simulink model "PI_Laengsregler"  (R2019b)
settings: Solver=FixedStepAuto  StartTime=0.0  StopTime=20  FixedStep=1e-6  RelTol=1e-3
values from neighbouring files (symbols this model uses):
  A = [0, 1;-f(1), -f(2)]    [init.m]    (also in matlab.mat = [0  1; -39.4784176044  -8.88576587632])
  b = [0; 1]    [init.m]    (also in matlab.mat = [0 1])
  cT = [f(1), 0]    [init.m]    (also in matlab.mat = [39.4784176044 0])
  ir = 1.7    [init.m]    (also in matlab.mat)
  pr = 1.3    [init.m]    (also in matlab.mat)
  tau = 3.215/5    (= 0.643)    [init.m]    (also in matlab.mat)
  Ur = pi*0.056    (= 0.175929188601)    [init.m]    (also in matlab.mat)
  v = 2    [init.m]    (also in matlab.mat)
libraries: robotlib x4, simulink x1, cstblocks x1

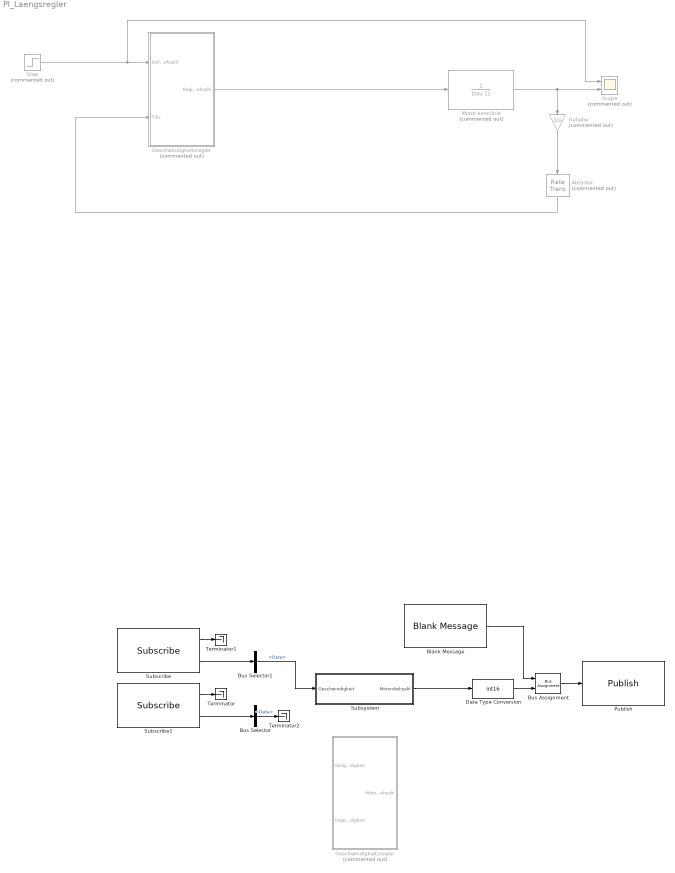
== system PI_Laengsregler ==
  Abtaster : RateTransition  Commented=on  OutPortSampleTime=tasten
  Blank Message : robotlib/Blank Message  messageClass=Message  entityType=std_msgs/Int16  messageType=std_msgs/Int16  SampleTime=inf
  Bus Assignment : BusAssignment  AssignedSignals=Data
  Bus Selector : BusSelector  OutputSignals=Data
  Bus Selector1 : BusSelector  OutputSignals=Data
  Data Type Conversion : DataTypeConversion  OutDataTypeStr=int16
  Geschwindigkeitsregler : Subsystem  Commented=on
  "Geschwindigkeitsregler " : Subsystem  Commented=on
  Getiebe : Gain  Commented=on  Gain=1/u
  Motor kennlinie : TransferFcn  Commented=on  Denominator=[tau 1]
  Publish : robotlib/Publish  topicSource=Specify your own  topic=/ctl_motorRpm  messageType=std_msgs/Int16  messageQueueLength=1
  Scope : Scope  Commented=on  NumInputPorts=2
  Step : Step  Commented=on  After=u*v/Ur  SampleTime=0
  Subscribe : robotlib/Subscribe  topicSource=Specify your own  topic=/trj_targetSpeed  messageType=std_msgs/Float32  sampleTime=-1  messageQueueLength=1
  Subscribe1 : robotlib/Subscribe  topicSource=Specify your own  topic=/ctl_velocity  messageType=std_msgs/Float32  sampleTime=-1  messageQueueLength=1
  Subsystem : Subsystem
  Terminator : Terminator
  Terminator1 : Terminator
  Terminator2 : Terminator
  wires:
  Getiebe/1 -> Abtaster/1
  Motor kennlinie/1 -> Getiebe/1, Scope/2
  Step/1 -> Scope/1, "Geschwindigkeitsregler "/1("Sollmotordrehzahl ")
  "Geschwindigkeitsregler "/1(Reglermotordrehzahl) -> Motor kennlinie/1
  Abtaster/1 -> "Geschwindigkeitsregler "/2(Tiks)
  Subscribe/2 -> Bus Selector1/1
  Subscribe1/2 -> Bus Selector/1
  Bus Assignment/1 -> Publish/1
  Blank Message/1 -> Bus Assignment/1
  Data Type Conversion/1 -> Bus Assignment/2
  Subscribe1/1 -> Terminator/1
  Subscribe/1 -> Terminator1/1
  Bus Selector1/1 -> Subsystem/1(Geschwindigkeit)  "<Data>"
  Subsystem/1(Motordrehzahl) -> Data Type Conversion/1
  Bus Selector/1 -> Terminator2/1  "<Data>"

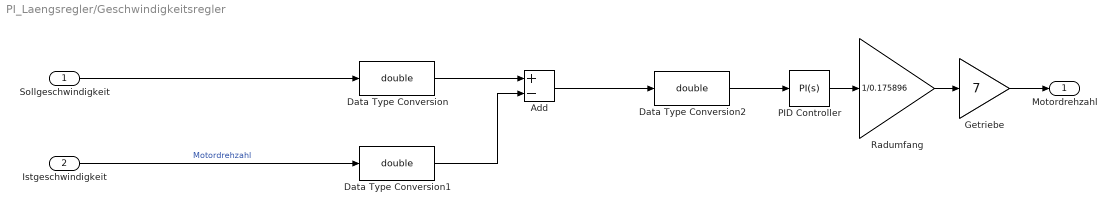
== system PI_Laengsregler/Geschwindigkeitsregler ==
  "Sollgeschwindigkeit " : Inport
  "Istgeschwindigkeit " : Inport  Port=2
  Add : Sum  Inputs=+-
  Data Type Conversion : DataTypeConversion  OutDataTypeStr=double
  Data Type Conversion1 : DataTypeConversion  OutDataTypeStr=double
  Data Type Conversion2 : DataTypeConversion  OutDataTypeStr=double
  Getriebe : Gain  Gain=7
  PID Controller : simulink/Continuous/PID Controller  Controller=PI  Form=Parallel  TimeDomain=Continuous-time  SampleTime=-1  IntegratorMethod=Forward Euler  FilterMethod=Forward Euler  ControllerParametersSource=internal  P=pr  I=ir  D=0  UseFilter=on  N=100  TunerSelectOption=Transfer Function Based (PID Tuner App)  InitialConditionSource=internal  InitialConditionForIntegrator=0  InitialConditionForFilter=0  DifferentiatorICPrevScaledInput=0  ExternalReset=none  TrackingMode=off  Kt=1  LimitOutput=off  UpperSaturationLimit=inf  LowerSaturationLimit=-inf  LinearizeAsGain=on  AntiWindupMode=none  Kb=1  POutMin=[]  POutMax=[]  IOutMin=[]  IOutMax=[]  DOutMin=[]  DOutMax=[]  NOutMin=[]  NOutMax=[]  SumOutMin=[]  SumOutMax=[]  SaturationOutMin=[]  SaturationOutMax=[]  PParamMin=[]  PParamMax=[]  IParamMin=[]  IParamMax=[]  DParamMin=[]  DParamMax=[]  NParamMin=[]  NParamMax=[]  KbParamMin=[]  KbParamMax=[]  KtParamMin=[]  KtParamMax=[]  KbOutMin=[]  KbOutMax=[]  KtOutMin=[]  KtOutMax=[]  IntegratorOutMin=[]  IntegratorOutMax=[]  FilterOutMin=[]  FilterOutMax=[]  SumI1OutMin=[]  SumI1OutMax=[]  SumI2OutMin=[]  SumI2OutMax=[]  SumI3OutMin=[]  SumI3OutMax=[]  SumI4OutMin=[]  SumI4OutMax=[]  SumDOutMin=[]  SumDOutMax=[]  DifferentiatorOutMin=[]  DifferentiatorOutMax=[]  FilterDiffOutCoefMin=[]  FilterDiffOutCoefMax=[]  ReciprocalOutMin=[]  ReciprocalOutMax=[]  SumDenOutMin=[]  SumDenOutMax=[]  SumNumOutMin=[]  SumNumOutMax=[]  DivideOutMin=[]  DivideOutMax=[]  IntegratorContinuousStateAttributes=''  IntegratorStateMustResolveToSignalObject=off  IntegratorRTWStateStorageClass=Auto  FilterContinuousStateAttributes=''  FilterStateMustResolveToSignalObject=off  FilterRTWStateStorageClass=Auto  ParallelPVariant=InternalParameters  IdealPVariant=Disabled  IVariant=InternalParameters  DVariant=Disabled  IntegratorVariant=Continuous  SatVariant=Disabled  AWVariant=Passthrough  PCopyVariant=Disabled  TRVariant=Disabled  FdbkBlocksVariant=Forward  IdealPFdbkVariant=Disabled  SatFdbkVariant=Disabled  DerivativeFilterVariant=Disabled  NVariant=Disabled  NCopyVariant=Disabled_SignalSpec  FilterICVariant=Disabled  IntegratorICVariant=InternalICs  ExternalResetVariant=Disabled  TRSumVariant=Passthrough  SumFdbkVariant=Disabled  SumVariant=Sum_PI
  Radumfang : Gain  Gain=1/0.175896
  "Motordrehzahl " : Outport
  wires:
  Add/1 -> Data Type Conversion2/1
  "Sollgeschwindigkeit "/1 -> Data Type Conversion/1
  PID Controller/1 -> Radumfang/1
  Data Type Conversion2/1 -> PID Controller/1
  Data Type Conversion1/1 -> Add/2
  Data Type Conversion/1 -> Add/1
  "Istgeschwindigkeit "/1 -> Data Type Conversion1/1  "Motordrehzahl"
  Radumfang/1 -> Getriebe/1
  Getriebe/1 -> "Motordrehzahl "/1

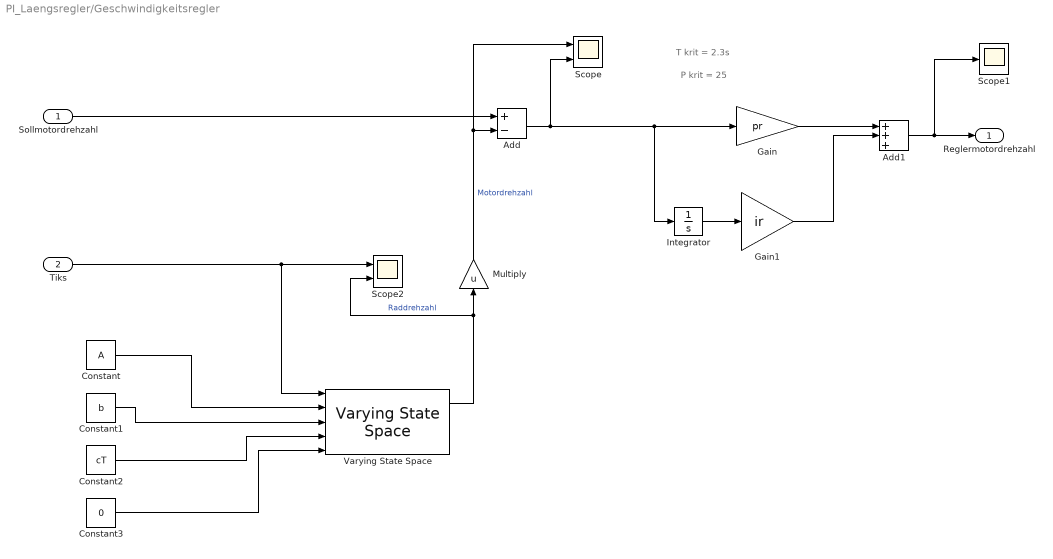
== system PI_Laengsregler/Geschwindigkeitsregler  ==
  note: T krit = 2.3s
  note: P krit = 25
  "Sollmotordrehzahl " : Inport
  Tiks : Inport  Port=2
  Add : Sum  Inputs=+-
  Add1 : Sum  Inputs=+++
  Constant : Constant  Value=A  VectorParams1D=off
  Constant1 : Constant  Value=b  VectorParams1D=off
  Constant2 : Constant  Value=cT  VectorParams1D=off
  Constant3 : Constant  Value=0
  Gain : Gain  Gain=pr
  Gain1 : Gain  Gain=ir
  Integrator : Integrator
  Multiply : Gain  Gain=u
  Scope : Scope  NumInputPorts=2
  Scope1 : Scope
  Scope2 : Scope  NumInputPorts=2
  Varying State Space : cstblocks/Linear Parameter Varying/Varying State Space  x0=0  xNames=''  OutputX=on  OutputDX=on
  Reglermotordrehzahl : Outport
  wires:
  Constant2/1 -> Varying State Space/4
  Integrator/1 -> Gain1/1
  Constant3/1 -> Varying State Space/5
  Constant1/1 -> Varying State Space/3
  Gain1/1 -> Add1/2
  Gain/1 -> Add1/1
  Varying State Space/1 -> Scope2/2, Multiply/1  "Raddrehzahl"
  Constant/1 -> Varying State Space/2
  Add1/1 -> Scope1/1, Reglermotordrehzahl/1
  Multiply/1 -> Scope/1, Add/2  "Motordrehzahl"
  Add/1 -> Scope/2, Integrator/1, Gain/1
  "Sollmotordrehzahl "/1 -> Add/1
  Tiks/1 -> Scope2/1, Varying State Space/1

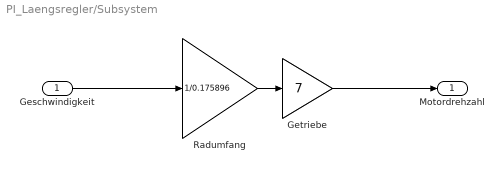
== system PI_Laengsregler/Subsystem ==
  Geschwindigkeit : Inport
  Getriebe : Gain  Gain=7
  Radumfang : Gain  Gain=1/0.175896
  Motordrehzahl : Outport
  wires:
  Radumfang/1 -> Getriebe/1
  Getriebe/1 -> Motordrehzahl/1
  Geschwindigkeit/1 -> Radumfang/1
